simulink model "F16TestHarness"  (R2024a)
settings: configuration reference "standardSILConfiguraitonParams" (kept outside this file)
undefined symbols (not defined in the file): airDensity_kgpm3, Earth, referenceLatitude_deg, referenceLongitude_deg, speedOfSound_mps, terrainHeightNED_m, visualizationType, WGS84
libraries: aerolibtransform2 x2, aerolibatmos2 x1, aerolibfltsims x1, sharedtransform x1, robotcorelib x1, uavutilslib x1
settings Model: Creator=jerem  LastModifiedBy=jerem
settings ConfigSetRef: SourceName=standardSILConfiguraitonParams  SourceLocation=Base Workspace

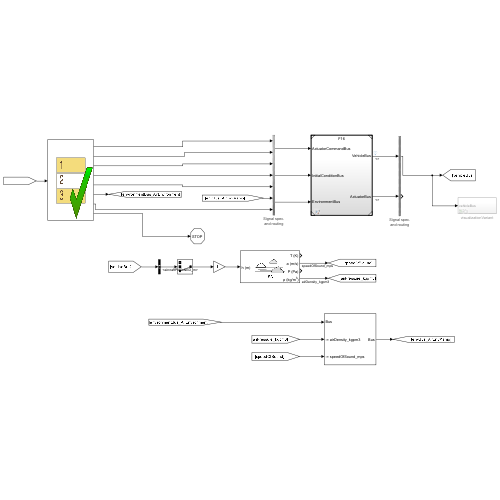
[thumbnail: Simulink's stored preview of the top-level diagram]
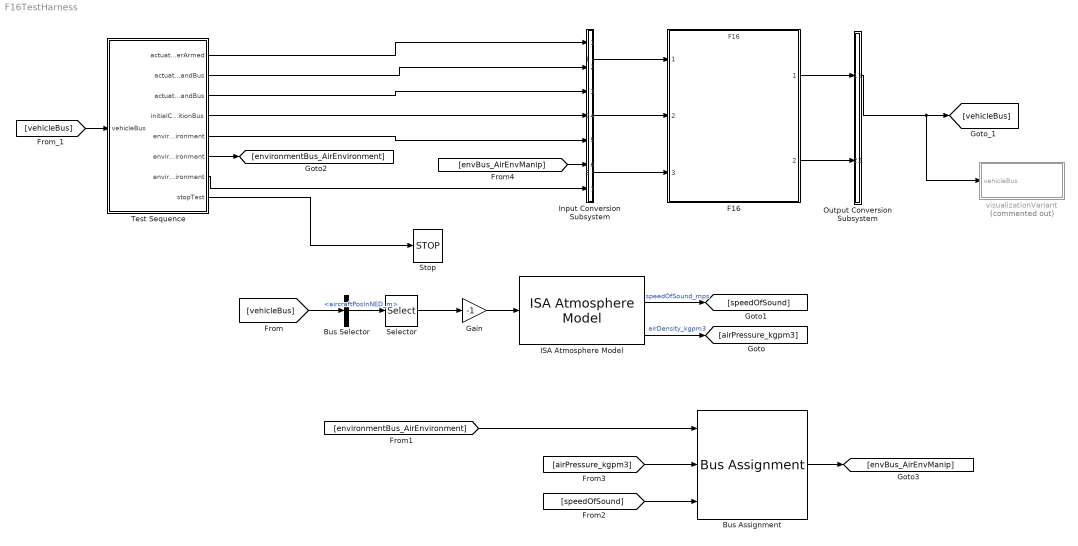
== system F16TestHarness ==
  Bus Assignment : BusAssignment  AssignedSignals=airDensity_kgpm3,speedOfSound_mps
  Bus Selector : BusSelector  OutputSignals=BodyStates.aircraftPosInNED_m
  F16 : ModelReference  ModelNameDialog=F16  SimulationMode=Normal  ModelReferenceVersion=1.92
  Gain : Gain  Gain=-1
  ISA Atmosphere Model : aerolibatmos2/ISA Atmosphere Model  useExtended=off  action=Warning  custom=off  viscosityOut=off  g=9.80665  gamma=1.4  R=287.0531  L=0.0065  h_trop=11000  h_strat=20000  rho0=1.225  P0=101325  T0=288.15  h0=0  S=110.4  Tref=273.15  muref=1.716e-5
  Input Conversion Subsystem : Subsystem  Tag=__SLT_ICS__  Description=|
      | Signal spec.
      | and routing
      settings: AttributesFormatString=%<Description>
  Output Conversion Subsystem : Subsystem  Tag=__SLT_OCS__  Description=|
      | Signal spec.
      | and routing
      mask init:
      | ICDictionary = get_param(bdroot, 'DataDictionary');
      | if isempty(ICDictionary)
      |    ICScope = Simulink.data.BaseWorkspace;
      | else
      |    ICScope = Simulink.data.DataDictionary(ICDictionary);
      | end
      | 
      | IC1 = Simulink.Bus.createMATLABStruct('VehicleBus', [], [1 1], ICScope);
      | IC2 = Simulink.Bus.createMATLABStruct('ActuatorBus', [], [1 1], ICScope);
      settings: AttributesFormatString=%<Description>
  Selector : Selector  InputPortWidth=3  IndexOptions=Index vector (dialog)  Indices=3  OutputSizes=1
  Stop : Stop
  Test Sequence : Test Sequence  TreatAsAtomicUnit=on
  visualizationVariant : Subsystem  Commented=on  Variant=on
  wires:
  Test Sequence/1(actuatorCommandBus_controllerArmed) -> Input Conversion Subsystem/1(Inport_1)
  Test Sequence/2(actuatorCommandBus_ServosCommandBus) -> Input Conversion Subsystem/2(Inport_2)
  Test Sequence/3(actuatorCommandBus_EngineCommandBus) -> Input Conversion Subsystem/3(Inport_3)
  Test Sequence/4(initialConditionBus) -> Input Conversion Subsystem/4(Inport_4)
  Test Sequence/5(environmentBus_EarthEnvironment) -> Input Conversion Subsystem/5(Inport_5)
  Test Sequence/6(environmentBus_AirEnvironment) -> [environmentBus_AirEnvironment]
  Test Sequence/7(environmentBus_TerrainEnvironment) -> Input Conversion Subsystem/7(Inport_7)
  [vehicleBus] -> Test Sequence/1(vehicleBus)
  Output Conversion Subsystem/1(Outport_1) -> visualizationVariant/1(vehicleBus), [vehicleBus]
  Test Sequence/8(stopTest) -> Stop/1
  [vehicleBus] -> Bus Selector/1
  Selector/1 -> Gain/1
  Bus Selector/1 -> Selector/1  "<aircraftPosInNED_m>"
  Gain/1 -> ISA Atmosphere Model/1
  ISA Atmosphere Model/4 -> [airPressure_kgpm3]  "airDensity_kgpm3"
  ISA Atmosphere Model/2 -> [speedOfSound]  "speedOfSound_mps"
  [environmentBus_AirEnvironment] -> Bus Assignment/1
  [speedOfSound] -> Bus Assignment/3
  [airPressure_kgpm3] -> Bus Assignment/2
  Bus Assignment/1 -> [envBus_AirEnvManip]
  [envBus_AirEnvManip] -> Input Conversion Subsystem/6(Inport_6)
  F16/1 -> Output Conversion Subsystem/1(Inport_1)
  F16/2 -> Output Conversion Subsystem/2(Inport_2)
  Input Conversion Subsystem/1(Outport_1) -> F16/1
  Input Conversion Subsystem/2(Outport_2) -> F16/2
  Input Conversion Subsystem/3(Outport_3) -> F16/3

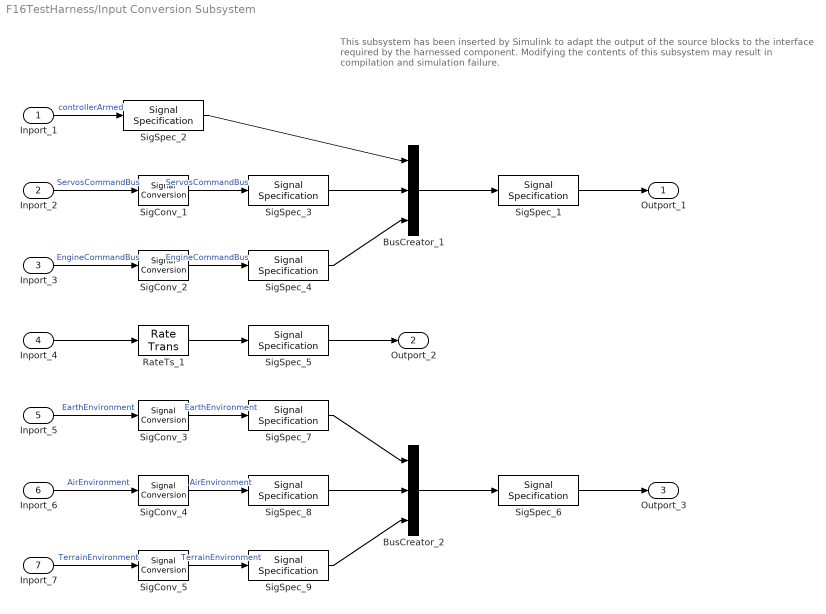
== system F16TestHarness/Input Conversion Subsystem ==
  note: This subsystem has been inserted by Simulink to adapt the output of the source blocks to the interface required by the harnessed component.
      |  Modifying the contents of this subsystem may result in compilation and simulation failure.
  Inport_1 : Inport
  Inport_2 : Inport  Port=2
  Inport_3 : Inport  Port=3
  Inport_4 : Inport  Port=4
  Inport_5 : Inport  Port=5
  Inport_6 : Inport  Port=6
  Inport_7 : Inport  Port=7
  BusCreator_1 : BusCreator  Inputs=3  OutDataTypeStr=Bus: ActuatorCommandBus
  BusCreator_2 : BusCreator  Inputs=3  OutDataTypeStr=Bus: EnvironmentBus
  RateTs_1 : RateTransition  OutPortSampleTime=0.004
  SigConv_{1..5} (5 alike) : SignalConversion  ConversionOutput=Nonvirtual bus  OverrideOpt=off
  SigSpec_1 : SignalSpecification  OutDataTypeStr=Bus: ActuatorCommandBus  SampleTime=[-1, 0]
  SigSpec_2 : SignalSpecification  OutDataTypeStr=double  Dimensions=[1]  SampleTime=[-1, 0]
  SigSpec_3 : SignalSpecification  OutDataTypeStr=Bus: ServosCommandBus  Dimensions=[1]  SampleTime=[-1, 0]  BusOutputAsStruct=on
  SigSpec_4 : SignalSpecification  OutDataTypeStr=Bus: EngineCommandBus  Dimensions=[1]  SampleTime=[-1, 0]  BusOutputAsStruct=on
  SigSpec_5 : SignalSpecification  OutDataTypeStr=double  Dimensions=[1]  SampleTime=0.004
  SigSpec_6 : SignalSpecification  OutDataTypeStr=Bus: EnvironmentBus  SampleTime=[-1, 0]
  SigSpec_7 : SignalSpecification  OutDataTypeStr=Bus: EarthEnvironmentBus  Dimensions=[1]  SampleTime=[-1, 0]  BusOutputAsStruct=on
  SigSpec_8 : SignalSpecification  OutDataTypeStr=Bus: AirEnvironmentBus  Dimensions=[1]  SampleTime=[-1, 0]  BusOutputAsStruct=on
  SigSpec_9 : SignalSpecification  OutDataTypeStr=Bus: TerrainEnvironmentBus  Dimensions=[1]  SampleTime=[-1, 0]  BusOutputAsStruct=on
  Outport_1 : Outport
  Outport_2 : Outport  Port=2
  Outport_3 : Outport  Port=3
  wires:
  SigSpec_1/1 -> Outport_1/1
  BusCreator_1/1 -> SigSpec_1/1
  SigSpec_2/1 -> BusCreator_1/1
  Inport_1/1 -> SigSpec_2/1  "controllerArmed"
  SigSpec_3/1 -> BusCreator_1/2
  SigConv_1/1 -> SigSpec_3/1  "ServosCommandBus"
  Inport_2/1 -> SigConv_1/1  "ServosCommandBus"
  SigSpec_4/1 -> BusCreator_1/3
  SigConv_2/1 -> SigSpec_4/1  "EngineCommandBus"
  Inport_3/1 -> SigConv_2/1  "EngineCommandBus"
  SigSpec_5/1 -> Outport_2/1
  RateTs_1/1 -> SigSpec_5/1
  Inport_4/1 -> RateTs_1/1
  SigSpec_6/1 -> Outport_3/1
  BusCreator_2/1 -> SigSpec_6/1
  SigSpec_7/1 -> BusCreator_2/1
  SigConv_3/1 -> SigSpec_7/1  "EarthEnvironment"
  Inport_5/1 -> SigConv_3/1  "EarthEnvironment"
  SigSpec_8/1 -> BusCreator_2/2
  SigConv_4/1 -> SigSpec_8/1  "AirEnvironment"
  Inport_6/1 -> SigConv_4/1  "AirEnvironment"
  SigSpec_9/1 -> BusCreator_2/3
  SigConv_5/1 -> SigSpec_9/1  "TerrainEnvironment"
  Inport_7/1 -> SigConv_5/1  "TerrainEnvironment"

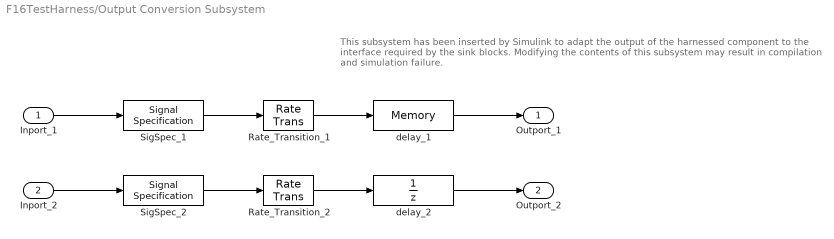
== system F16TestHarness/Output Conversion Subsystem ==
  note: This subsystem has been inserted by Simulink to adapt the output of the harnessed component to the interface required by the sink blocks.
      |  Modifying the contents of this subsystem may result in compilation and simulation failure.
  Inport_1 : Inport
  Inport_2 : Inport  Port=2
  Rate_Transition_1 : RateTransition  OutPortSampleTimeOpt=Inherit
  Rate_Transition_2 : RateTransition  OutPortSampleTimeOpt=Inherit
  SigSpec_1 : SignalSpecification  OutDataTypeStr=Bus: VehicleBus  Dimensions=[1]
  SigSpec_2 : SignalSpecification  OutDataTypeStr=Bus: ActuatorBus  Dimensions=[1]
  delay_1 : Memory  InitialCondition=IC1
  delay_2 : UnitDelay  InitialCondition=IC2  SampleTime=-1
  Outport_1 : Outport
  Outport_2 : Outport  Port=2
  wires:
  Inport_1/1 -> SigSpec_1/1
  SigSpec_1/1 -> Rate_Transition_1/1
  Rate_Transition_1/1 -> delay_1/1
  delay_1/1 -> Outport_1/1
  Inport_2/1 -> SigSpec_2/1
  SigSpec_2/1 -> Rate_Transition_2/1
  Rate_Transition_2/1 -> delay_2/1
  delay_2/1 -> Outport_2/1

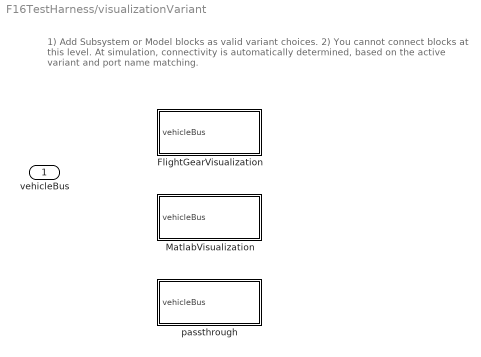
== system F16TestHarness/visualizationVariant ==
  note: 1) Add Subsystem or Model blocks as valid variant choices.
      | 2) You cannot connect blocks at this level. At simulation, connectivity is automatically
      | determined, based on the active variant and port name matching.
  vehicleBus : Inport
  FlightGearVisualization : Subsystem  TreatAsAtomicUnit=on  VariantControl="strcmp(visualizationType, \"FlightGear\")"
  MatlabVisualization : Subsystem  VariantControl="strcmp(visualizationType, \"Matlab\")"
  passthrough : Subsystem  VariantControl="strcmp(visualizationType, \"PassThrough\")"

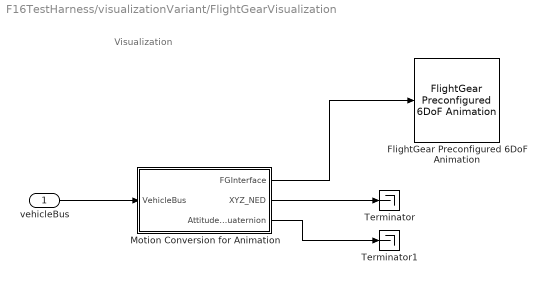
== system F16TestHarness/visualizationVariant/FlightGearVisualization ==
  note: Visualization
  vehicleBus : Inport
  FlightGear Preconfigured 6DoF Animation : aerolibfltsims/FlightGear Preconfigured 6DoF Animation  xFlightGearVersion=v2019.1  DestinationIpAddress=127.0.0.1  DestinationPort=5502  SampleTime=-1  packetVersion=24
  Motion Conversion for Animation : Subsystem
      mask Display:
      | port_label('input',1,'ACBus')
      | port_label('output',1,'\lambda,L,h,\phi,\theta,\psi','texmode','on')
  Terminator : Terminator
  Terminator1 : Terminator
  wires:
  Motion Conversion for Animation/1(FGInterface) -> FlightGear Preconfigured 6DoF Animation/1
  vehicleBus/1 -> Motion Conversion for Animation/1(VehicleBus)
  Motion Conversion for Animation/2(XYZ_NED) -> Terminator/1
  Motion Conversion for Animation/3(AttitudeQuaternion) -> Terminator1/1

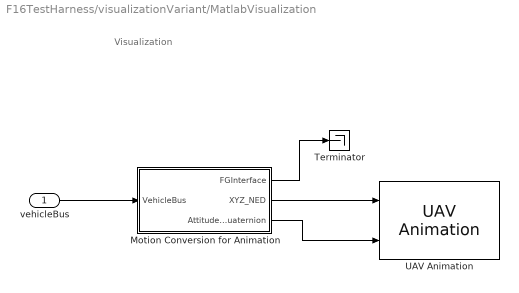
== system F16TestHarness/visualizationVariant/MatlabVisualization ==
  note: Visualization
  vehicleBus : Inport
  Motion Conversion for Animation : Subsystem
      mask Display:
      | port_label('input',1,'ACBus')
      | port_label('output',1,'\lambda,L,h,\phi,\theta,\psi','texmode','on')
  Terminator : Terminator
  UAV Animation : uavutilslib/UAV Animation  UAVType=FixedWing  UAVSize=100  InertialZDirection=Down  SampleTime=-1
  wires:
  Motion Conversion for Animation/2(XYZ_NED) -> UAV Animation/1
  vehicleBus/1 -> Motion Conversion for Animation/1(VehicleBus)
  Motion Conversion for Animation/3(AttitudeQuaternion) -> UAV Animation/2
  Motion Conversion for Animation/1(FGInterface) -> Terminator/1

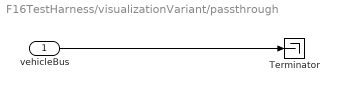
== system F16TestHarness/visualizationVariant/passthrough ==
  vehicleBus : Inport
  Terminator : Terminator
  wires:
  vehicleBus/1 -> Terminator/1

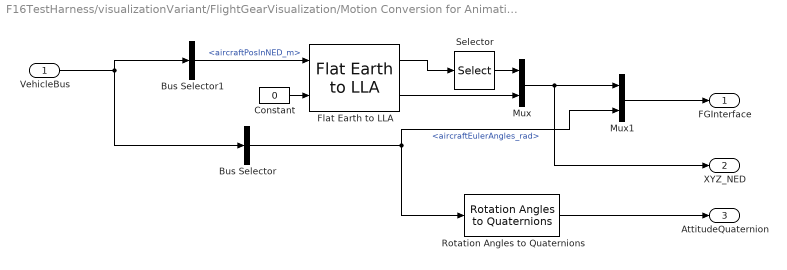
== system F16TestHarness/visualizationVariant/FlightGearVisualization/Motion Conversion for Animation ==
  VehicleBus : Inport  OutDataTypeStr=Bus: VehicleBus
  Bus Selector : BusSelector  OutputSignals=BodyStates.aircraftEulerAngles_rad
  Bus Selector1 : BusSelector  OutputSignals=BodyStates.aircraftPosInNED_m
  Constant : Constant  Value=0
  Flat Earth to LLA : aerolibtransform2/Flat Earth to LLA  units=Metric (MKS)  ptype=Earth (WGS84)  F=1/298.257223563  R=6378137  refPosPort=off  LL0=[referenceLatitude_deg, referenceLongitude_deg]  psi=0
  Mux : Mux  Inputs=2
  Mux1 : Mux  Inputs=2
  Rotation Angles to Quaternions : sharedtransform/Rotation Angles to Quaternions  rotationOrder=ZYX  aMode=aMode
  Selector : Selector  IndexMode=Zero-based  InputPortWidth=2  IndexOptions=Index vector (dialog)  Indices=[1 0]  OutputSizes=1
  FGInterface : Outport  VectorParamsAs1DForOutWhenUnconnected=off
  XYZ_NED : Outport  Port=2  VectorParamsAs1DForOutWhenUnconnected=off
  AttitudeQuaternion : Outport  Port=3  VectorParamsAs1DForOutWhenUnconnected=off
  wires:
  Mux1/1 -> FGInterface/1
  Constant/1 -> Flat Earth to LLA/2
  Bus Selector/1 -> Rotation Angles to Quaternions/1, Mux1/2  "<aircraftEulerAngles_rad>"
  Flat Earth to LLA/2 -> Mux/2
  Flat Earth to LLA/1 -> Selector/1
  Bus Selector1/1 -> Flat Earth to LLA/1  "<aircraftPosInNED_m>"
  VehicleBus/1 -> Bus Selector/1, Bus Selector1/1
  Selector/1 -> Mux/1
  Mux/1 -> XYZ_NED/1, Mux1/1
  Rotation Angles to Quaternions/1 -> AttitudeQuaternion/1

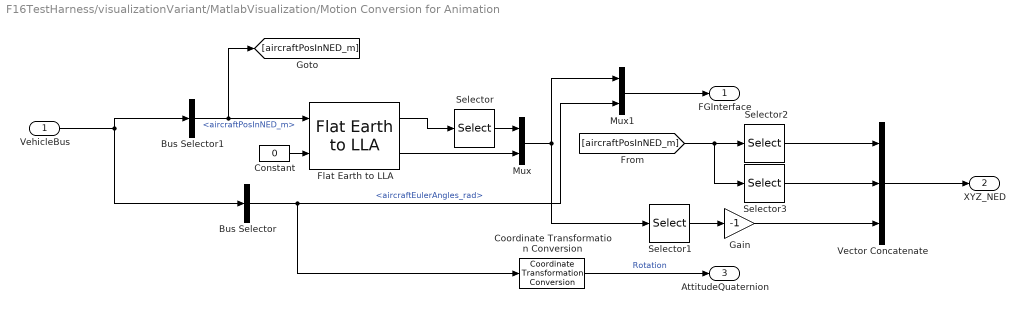
== system F16TestHarness/visualizationVariant/MatlabVisualization/Motion Conversion for Animation ==
  VehicleBus : Inport  OutDataTypeStr=Bus: VehicleBus
  Bus Selector : BusSelector  OutputSignals=BodyStates.aircraftEulerAngles_rad
  Bus Selector1 : BusSelector  OutputSignals=BodyStates.aircraftPosInNED_m
  Constant : Constant  Value=0
  Coordinate Transformation Conversion : robotcorelib/Coordinate Transformation Conversion  InputRepresentation=Euler Angles  InputEulerSequence=XYZ  ShowTrVecInputPort=on  OutputRepresentation=Quaternion  OutputEulerSequence=ZYX  ShowTrVecOutputPort=on  SimulateUsing=Code generation
  Flat Earth to LLA : aerolibtransform2/Flat Earth to LLA  units=Metric (MKS)  ptype=Earth (WGS84)  F=1/298.257223563  R=6378137  refPosPort=off  LL0=[referenceLatitude_deg, referenceLongitude_deg]  psi=0
  Gain : Gain  Gain=-1
  Mux : Mux  Inputs=2
  Mux1 : Mux  Inputs=2
  Selector : Selector  IndexMode=Zero-based  InputPortWidth=2  IndexOptions=Index vector (dialog)  Indices=[1 0]  OutputSizes=1
  Selector1 : Selector  InputPortWidth=3  IndexOptions=Index vector (dialog)  Indices=3  OutputSizes=1
  Selector2 : Selector  InputPortWidth=3  IndexOptions=Index vector (dialog)  Indices=1  OutputSizes=1
  Selector3 : Selector  InputPortWidth=3  IndexOptions=Index vector (dialog)  Indices=2  OutputSizes=1
  Vector Concatenate : Concatenate  NumInputs=3
  FGInterface : Outport  VectorParamsAs1DForOutWhenUnconnected=off
  XYZ_NED : Outport  Port=2  VectorParamsAs1DForOutWhenUnconnected=off
  AttitudeQuaternion : Outport  Port=3  VectorParamsAs1DForOutWhenUnconnected=off
  wires:
  Mux1/1 -> FGInterface/1
  Constant/1 -> Flat Earth to LLA/2
  Bus Selector/1 -> Coordinate Transformation Conversion/1, Mux1/2  "<aircraftEulerAngles_rad>"
  Flat Earth to LLA/2 -> Mux/2
  Flat Earth to LLA/1 -> Selector/1
  Bus Selector1/1 -> [aircraftPosInNED_m], Flat Earth to LLA/1  "<aircraftPosInNED_m>"
  VehicleBus/1 -> Bus Selector/1, Bus Selector1/1
  Selector/1 -> Mux/1
  Mux/1 -> Selector1/1, Mux1/1
  Selector2/1 -> Vector Concatenate/1
  Selector3/1 -> Vector Concatenate/2
  Vector Concatenate/1 -> XYZ_NED/1
  Selector1/1 -> Gain/1
  Gain/1 -> Vector Concatenate/3
  [aircraftPosInNED_m] -> Selector3/1, Selector2/1
  Coordinate Transformation Conversion/1 -> AttitudeQuaternion/1  "Rotation"

== stateflow chart F16TestHarness/Test Sequence ==
  state Scenario_1
    state Initialize
      %% Initialize data outputs.
      actuatorCommandBus_controllerArmed = 0;
      actuatorCommandBus_ServosCommandBus.ServosCommandF16Bus.cmdAileron_nd = 0;
      actuatorCommandBus_ServosCommandBus.ServosCommandF16Bus.cmdElevator_nd = 0;
      actuatorCommandBus_ServosCommandBus.ServosCommandF16Bus.cmdRudder_nd = 0;
      actuatorCommandBus_EngineCommandBus.cmdThrottle_unit = 0;
      initialConditionBus = 0;
      environmentBus_EarthEnvironment.gravityScalar_mps2 = 9.80665;
      environmentBus_EarthEnvironment.worldMagneticFieldInNED_nT = zeros(3,1);
      environmentBus_AirEnvironment.airTemperature_K = 0;
      environmentBus_AirEnvironment.airPressure_Pa = 0;
      environmentBus_AirEnvironment.airDensity_kgpm3 = 1.225;
      environmentBus_AirEnvironment.windSpeedInNED_mps = zeros(3,1);
      environmentBus_AirEnvironment.speedOfSound_mps = 0;
      environmentBus_AirEnvironment.windsAloftInNED_mps = zeros(3,1);
      environmentBus_AirEnvironment.gustInNED_mps = zeros(3,1);
      environmentBus_AirEnvironment.turbulenceInNED_mps = zeros(3,1);
      environmentBus_TerrainEnvironment.terrainHeightInNED_m = terrainHeightNED_m;
      stopTest = false;
    state verifyZeroInputs
      verify(isClose(vehicleBus.AircraftForcesMoments.forcesInBody_N(1), 0 ))
      verify(isClose(vehicleBus.AircraftForcesMoments.forcesInBody_N(2), 0 ))
      verify(isClose(vehicleBus.AircraftForcesMoments.forcesInBody_N(3), 0 ))
      verify(isClose(vehicleBus.AircraftForcesMoments.momentsInBody_Nm(1),0))
      verify(isClose(vehicleBus.AircraftForcesMoments.momentsInBody_Nm(2),0))
      verify(isClose(vehicleBus.AircraftForcesMoments.momentsInBody_Nm(3),0))
    state throttleNoArm
      actuatorCommandBus_EngineCommandBus.cmdThrottle_unit = 0.1;
    state noThrottleArm
      actuatorCommandBus_controllerArmed = 1;
      actuatorCommandBus_EngineCommandBus.cmdThrottle_unit = 0.0;
      %actuatorCommandBus_ServosCommandBus.ServosCommandF16Bus.cmdElevator_nd = -0.1;
    state verifyZeroInputsAgain
      verify(isClose(vehicleBus.AircraftForcesMoments.forcesInBody_N(1), 0 ))
      verify(isClose(vehicleBus.AircraftForcesMoments.forcesInBody_N(2), 0 ))
      verify(isClose(vehicleBus.AircraftForcesMoments.forcesInBody_N(3), 0 ))
      verify(isClose(vehicleBus.AircraftForcesMoments.momentsInBody_Nm(1),0))
      verify(isClose(vehicleBus.AircraftForcesMoments.momentsInBody_Nm(2),0))
      verify(isClose(vehicleBus.AircraftForcesMoments.momentsInBody_Nm(3),0))
    state armedAndSmallThrottle
      actuatorCommandBus_EngineCommandBus.cmdThrottle_unit = 0.25;
    state verifyThrottle
      verify(vehicleBus.AircraftForcesMoments.forcesInBody_N(1) > 0)
      verify(isClose(vehicleBus.AircraftForcesMoments.forcesInBody_N(2), 0 ))
      verify(isClose(vehicleBus.AircraftForcesMoments.forcesInBody_N(3), 0 ))
      verify(isClose(vehicleBus.AircraftForcesMoments.momentsInBody_Nm(1),0))
      verify(isClose(vehicleBus.AircraftForcesMoments.momentsInBody_Nm(2),0))
      verify(isClose(vehicleBus.AircraftForcesMoments.momentsInBody_Nm(3),0))
    state deflectElevatorCreatingNegPitch
      actuatorCommandBus_ServosCommandBus.ServosCommandF16Bus.cmdElevator_nd = 0.25;
      actuatorCommandBus_EngineCommandBus.cmdThrottle_unit = 0.75;
    state verifyPitchIntoGround
      verify(isClose(vehicleBus.AircraftForcesMoments.momentsInBody_Nm(2), 0))
      verify(isClose(vehicleBus.BodyStates.aircraftEulerAngles_rad(2) , 0))
      verify(isClose(vehicleBus.AircraftForcesMoments.forcesInBody_N(3), 0))
      verify(vehicleBus.AircraftForcesMoments.forcesInBody_N(1) > 0)
      verify(isClose(vehicleBus.AircraftForcesMoments.forcesInBody_N(2), 0 ))
    state deflectElevator
      actuatorCommandBus_ServosCommandBus.ServosCommandF16Bus.cmdElevator_nd = -0.025;
      actuatorCommandBus_EngineCommandBus.cmdThrottle_unit = 1;
    state verifydeflectElevator
      verify(isClose(vehicleBus.AircraftForcesMoments.momentsInBody_Nm(2), 0, 'absTol', 0.01)) % Shouldn't be enough elevator to rotate vehicle
      verify(isClose(vehicleBus.BodyStates.aircraftEulerAngles_rad(2), 0, 'absTol', 0.01 )) % Shouldn't be enough elevator to rotate vehicle
      verify(isClose(vehicleBus.AircraftForcesMoments.forcesInBody_N(3), 0, 'absTol', 0.01))
      verify(vehicleBus.AircraftForcesMoments.forcesInBody_N(1) > 0)
      verify(isClose(vehicleBus.AircraftForcesMoments.forcesInBody_N(2), 0 ))
    state rotate
      actuatorCommandBus_ServosCommandBus.ServosCommandF16Bus.cmdElevator_nd = -0.08;
    state verifyRotate
      verify(vehicleBus.AircraftForcesMoments.momentsInBody_Nm(2) > 0)
      verify(vehicleBus.BodyStates.aircraftEulerAngles_rad(2) > 0)
      verify(vehicleBus.AircraftForcesMoments.forcesInBody_N(3) < 0)
      verify(vehicleBus.AircraftForcesMoments.forcesInBody_N(1) > 0)
      verify(isClose(vehicleBus.AircraftForcesMoments.forcesInBody_N(2), 0 ))
    state continueFlying
      actuatorCommandBus_ServosCommandBus.ServosCommandF16Bus.cmdElevator_nd = -0.04;
      actuatorCommandBus_EngineCommandBus.cmdThrottle_unit = 1;
    state verifyFlying
      verify(vehicleBus.BodyStates.aircraftPosInNED_m(3) < 0)
      verify(vehicleBus.BodyStates.aircraftEulerAngles_rad(2) > 0)
      verify(vehicleBus.AircraftForcesMoments.forcesInBody_N(1) > 0)
      verify(isClose(vehicleBus.AircraftForcesMoments.forcesInBody_N(2), 0 ))
    state EndTest
      stopTest = true;
    (default) -> Scenario_1.Initialize
    Scenario_1.Initialize -> verifyZeroInputs : [
        | after(1,tick)
        | ]
    verifyZeroInputs -> throttleNoArm : [
        | after(5,sec)
        | ]
    throttleNoArm -> noThrottleArm : [
        | after(1,sec)
        | ]
    noThrottleArm -> verifyZeroInputsAgain : [
        | after(3,sec)
        | ]
    verifyZeroInputsAgain -> armedAndSmallThrottle : [
        | after(5,sec)
        | ]
    armedAndSmallThrottle -> verifyThrottle : [
        | after(60,sec)
        | ]
    verifyThrottle -> deflectElevatorCreatingNegPitch : [
        | after(1,tick)
        | ]
    deflectElevatorCreatingNegPitch -> verifyPitchIntoGround : [
        | after(3,sec)
        | ]
    verifyPitchIntoGround -> deflectElevator : [
        | after(1,sec)
        | ]
    deflectElevator -> verifydeflectElevator : [
        | after(2,sec)
        | ]
    verifydeflectElevator -> rotate : [
        | after(1,tick)
        | ]
    rotate -> verifyRotate : [
        | after(3,sec)
        | ]
    verifyRotate -> continueFlying : [
        | after(1,tick)
        | ]
    continueFlying -> verifyFlying : [
        | after(3,sec)
        | ]
    verifyFlying -> Scenario_1.EndTest : [
        | after(1,tick)
        | ]
  state SameAsVehiclePlantHarness
    state Initialize
      %% Initialize data outputs.
      actuatorCommandBus_controllerArmed = 0;
      actuatorCommandBus_ServosCommandBus.ServosCommandF16Bus.cmdAileron_nd = 0;
      actuatorCommandBus_ServosCommandBus.ServosCommandF16Bus.cmdElevator_nd = 0;
      actuatorCommandBus_ServosCommandBus.ServosCommandF16Bus.cmdRudder_nd = 0;
      actuatorCommandBus_EngineCommandBus.cmdThrottle_unit = 0;
      initialConditionBus = 0;
      environmentBus_EarthEnvironment.gravityScalar_mps2 = 9.80665;
      environmentBus_EarthEnvironment.worldMagneticFieldInNED_nT = zeros(3,1);
      environmentBus_AirEnvironment.airTemperature_K = 0;
      environmentBus_AirEnvironment.airPressure_Pa = 0;
      environmentBus_AirEnvironment.airDensity_kgpm3 = 1.225;
      environmentBus_AirEnvironment.windSpeedInNED_mps = zeros(3,1);
      environmentBus_AirEnvironment.speedOfSound_mps = 0;
      environmentBus_AirEnvironment.windsAloftInNED_mps = zeros(3,1);
      environmentBus_AirEnvironment.gustInNED_mps = zeros(3,1);
      environmentBus_AirEnvironment.turbulenceInNED_mps = zeros(3,1);
      environmentBus_TerrainEnvironment.terrainHeightInNED_m = terrainHeightNED_m;
      stopTest = false;
    state step_1
      actuatorCommandBus_controllerArmed = 1;
      actuatorCommandBus_ServosCommandBus.ServosCommandF16Bus.cmdElevator_nd = -0.15;
      actuatorCommandBus_EngineCommandBus.cmdThrottle_unit = 1;
    state step_2
      actuatorCommandBus_ServosCommandBus.ServosCommandF16Bus.cmdElevator_nd  = -0.03;
    state step_3
      actuatorCommandBus_ServosCommandBus.ServosCommandF16Bus.cmdElevator_nd  = -0.1;
    state EndTest
      stopTest = true;
    (default) -> SameAsVehiclePlantHarness.Initialize
    SameAsVehiclePlantHarness.Initialize -> SameAsVehiclePlantHarness.step_1 : [
        | after(1,tick)
        | ]
    SameAsVehiclePlantHarness.step_1 -> SameAsVehiclePlantHarness.step_2 : [
        | after(30,sec)
        | ]
    SameAsVehiclePlantHarness.step_2 -> SameAsVehiclePlantHarness.step_3 : [
        | after(100,sec)
        | ]
    SameAsVehiclePlantHarness.step_3 -> SameAsVehiclePlantHarness.EndTest : [
        | after(150,sec)
        | ]
  state MaxAirspeedTest
    state Initialize
      %% Initialize data outputs.
      actuatorCommandBus_controllerArmed = 0;
      actuatorCommandBus_ServosCommandBus.ServosCommandF16Bus.cmdAileron_nd = 0;
      actuatorCommandBus_ServosCommandBus.ServosCommandF16Bus.cmdElevator_nd = 0;
      actuatorCommandBus_ServosCommandBus.ServosCommandF16Bus.cmdRudder_nd = 0;
      actuatorCommandBus_EngineCommandBus.cmdThrottle_unit = 0;
      initialConditionBus = 0;
      environmentBus_EarthEnvironment.gravityScalar_mps2 = 9.80665;
      environmentBus_EarthEnvironment.worldMagneticFieldInNED_nT = zeros(3,1);
      environmentBus_AirEnvironment.airTemperature_K = 0;
      environmentBus_AirEnvironment.airPressure_Pa = 0;
      environmentBus_AirEnvironment.airDensity_kgpm3 = 1.225;
      environmentBus_AirEnvironment.windSpeedInNED_mps = zeros(3,1);
      environmentBus_AirEnvironment.speedOfSound_mps = 0;
      environmentBus_AirEnvironment.windsAloftInNED_mps = zeros(3,1);
      environmentBus_AirEnvironment.gustInNED_mps = zeros(3,1);
      environmentBus_AirEnvironment.turbulenceInNED_mps = zeros(3,1);
      environmentBus_TerrainEnvironment.terrainHeightInNED_m = terrainHeightNED_m;
      stopTest = false;
    state step_1
      actuatorCommandBus_controllerArmed = 1;
      actuatorCommandBus_ServosCommandBus.ServosCommandF16Bus.cmdElevator_nd = -0.05;
      actuatorCommandBus_EngineCommandBus.cmdThrottle_unit = 1;
    state step_2
      actuatorCommandBus_ServosCommandBus.ServosCommandF16Bus.cmdElevator_nd = 0;
    state EndTest
      stopTest = true;
    (default) -> MaxAirspeedTest.Initialize
    MaxAirspeedTest.Initialize -> MaxAirspeedTest.step_1 : [
        | after(1,tick)
        | ]
    MaxAirspeedTest.step_1 -> MaxAirspeedTest.step_2 : [
        | after(25,sec)
        | ]
    MaxAirspeedTest.step_2 -> MaxAirspeedTest.EndTest : [
        | after(200,sec)
        | ]
  state TakeoffLevelFlight
    state Initialize
      %% Initialize data outputs.
      actuatorCommandBus_controllerArmed = 0;
      actuatorCommandBus_ServosCommandBus.ServosCommandF16Bus.cmdAileron_nd = 0;
      actuatorCommandBus_ServosCommandBus.ServosCommandF16Bus.cmdElevator_nd = 0;
      actuatorCommandBus_ServosCommandBus.ServosCommandF16Bus.cmdRudder_nd = 0;
      actuatorCommandBus_EngineCommandBus.cmdThrottle_unit = 0;
      initialConditionBus = 0;
      environmentBus_EarthEnvironment.gravityScalar_mps2 = 9.80665;
      environmentBus_EarthEnvironment.worldMagneticFieldInNED_nT = zeros(3,1);
      environmentBus_AirEnvironment.airTemperature_K = 0;
      environmentBus_AirEnvironment.airPressure_Pa = 0;
      environmentBus_AirEnvironment.airDensity_kgpm3 = 1.225;
      environmentBus_AirEnvironment.windSpeedInNED_mps = zeros(3,1);
      environmentBus_AirEnvironment.speedOfSound_mps = 0;
      environmentBus_AirEnvironment.windsAloftInNED_mps = zeros(3,1);
      environmentBus_AirEnvironment.gustInNED_mps = zeros(3,1);
      environmentBus_AirEnvironment.turbulenceInNED_mps = zeros(3,1);
      environmentBus_TerrainEnvironment.terrainHeightInNED_m = terrainHeightNED_m;
      stopTest = false;
    state step_2
      actuatorCommandBus_controllerArmed = 1;
      actuatorCommandBus_EngineCommandBus.cmdThrottle_unit = 1;
    state step_3
      actuatorCommandBus_ServosCommandBus.ServosCommandF16Bus.cmdElevator_nd = -0.08;
    state step_1
      actuatorCommandBus_ServosCommandBus.ServosCommandF16Bus.cmdElevator_nd = -0.04;
    state step_4
      actuatorCommandBus_ServosCommandBus.ServosCommandF16Bus.cmdElevator_nd = -0.028;
    state EndTest
      stopTest = true;
    (default) -> TakeoffLevelFlight.Initialize
    TakeoffLevelFlight.Initialize -> TakeoffLevelFlight.step_2 : [
        | after(1,tick)
        | ]
    TakeoffLevelFlight.step_2 -> TakeoffLevelFlight.step_3 : [
        | after(22,sec)
        | ]
    TakeoffLevelFlight.step_3 -> TakeoffLevelFlight.step_1 : [
        | after(10,sec)
        | ]
    TakeoffLevelFlight.step_1 -> TakeoffLevelFlight.step_4 : [
        | after(20,sec)
        | ]
    TakeoffLevelFlight.step_4 -> TakeoffLevelFlight.EndTest : [
        | after(20,sec)
        | ]
  state pitchTest
    state Initialize
      %% Initialize data outputs.
      actuatorCommandBus_controllerArmed = 0;
      actuatorCommandBus_ServosCommandBus.ServosCommandF16Bus.cmdAileron_nd = 0;
      actuatorCommandBus_ServosCommandBus.ServosCommandF16Bus.cmdElevator_nd = 0;
      actuatorCommandBus_ServosCommandBus.ServosCommandF16Bus.cmdRudder_nd = 0;
      actuatorCommandBus_EngineCommandBus.cmdThrottle_unit = 0;
      initialConditionBus = 0;
      environmentBus_EarthEnvironment.gravityScalar_mps2 = 9.80665;
      environmentBus_EarthEnvironment.worldMagneticFieldInNED_nT = zeros(3,1);
      environmentBus_AirEnvironment.airTemperature_K = 0;
      environmentBus_AirEnvironment.airPressure_Pa = 0;
      environmentBus_AirEnvironment.airDensity_kgpm3 = 1.225;
      environmentBus_AirEnvironment.windSpeedInNED_mps = zeros(3,1);
      environmentBus_AirEnvironment.speedOfSound_mps = 0;
      environmentBus_AirEnvironment.windsAloftInNED_mps = zeros(3,1);
      environmentBus_AirEnvironment.gustInNED_mps = zeros(3,1);
      environmentBus_AirEnvironment.turbulenceInNED_mps = zeros(3,1);
      environmentBus_TerrainEnvironment.terrainHeightInNED_m = terrainHeightNED_m;
      stopTest = false;
    state step_2
      actuatorCommandBus_controllerArmed = 1;
      actuatorCommandBus_EngineCommandBus.cmdThrottle_unit = 1;
    state step_3
      actuatorCommandBus_ServosCommandBus.ServosCommandF16Bus.cmdElevator_nd = -0.08;
    state step_1
      actuatorCommandBus_ServosCommandBus.ServosCommandF16Bus.cmdElevator_nd = -0.04;
    state step_5
      actuatorCommandBus_ServosCommandBus.ServosCommandF16Bus.cmdElevator_nd = -1;
    state EndTest
      stopTest = true;
    (default) -> pitchTest.Initialize
    pitchTest.Initialize -> pitchTest.step_2 : [
        | after(1,tick)
        | ]
    pitchTest.step_2 -> pitchTest.step_3 : [
        | after(22,sec)
        | ]
    pitchTest.step_3 -> pitchTest.step_1 : [
        | after(10,sec)
        | ]
    pitchTest.step_5 -> pitchTest.EndTest : [
        | after(8,sec)
        | ]
    pitchTest.step_1 -> pitchTest.step_5 : [
        | after(20,sec)
        | ]
  state rollTest
    state Initialize
      %% Initialize data outputs.
      actuatorCommandBus_controllerArmed = 0;
      actuatorCommandBus_ServosCommandBus.ServosCommandF16Bus.cmdAileron_nd = 0;
      actuatorCommandBus_ServosCommandBus.ServosCommandF16Bus.cmdElevator_nd = 0;
      actuatorCommandBus_ServosCommandBus.ServosCommandF16Bus.cmdRudder_nd = 0;
      actuatorCommandBus_EngineCommandBus.cmdThrottle_unit = 0;
      initialConditionBus = 0;
      environmentBus_EarthEnvironment.gravityScalar_mps2 = 9.80665;
      environmentBus_EarthEnvironment.worldMagneticFieldInNED_nT = zeros(3,1);
      environmentBus_AirEnvironment.airTemperature_K = 0;
      environmentBus_AirEnvironment.airPressure_Pa = 0;
      environmentBus_AirEnvironment.airDensity_kgpm3 = 1.225;
      environmentBus_AirEnvironment.windSpeedInNED_mps = zeros(3,1);
      environmentBus_AirEnvironment.speedOfSound_mps = 0;
      environmentBus_AirEnvironment.windsAloftInNED_mps = zeros(3,1);
      environmentBus_AirEnvironment.gustInNED_mps = zeros(3,1);
      environmentBus_AirEnvironment.turbulenceInNED_mps = zeros(3,1);
      environmentBus_TerrainEnvironment.terrainHeightInNED_m = terrainHeightNED_m;
      stopTest = false;
    state step_2
      actuatorCommandBus_controllerArmed = 1;
      actuatorCommandBus_EngineCommandBus.cmdThrottle_unit = 1;
    state step_3
      actuatorCommandBus_ServosCommandBus.ServosCommandF16Bus.cmdElevator_nd = -0.08;
    state step_1
      actuatorCommandBus_ServosCommandBus.ServosCommandF16Bus.cmdElevator_nd = -0.04;
    state step_5
      actuatorCommandBus_ServosCommandBus.ServosCommandF16Bus.cmdAileron_nd= -1;
      actuatorCommandBus_ServosCommandBus.ServosCommandF16Bus.cmdElevator_nd = 0;
    state EndTest
      stopTest = true;
    (default) -> rollTest.Initialize
    rollTest.Initialize -> rollTest.step_2 : [
        | after(1,tick)
        | ]
    rollTest.step_2 -> rollTest.step_3 : [
        | after(22,sec)
        | ]
    rollTest.step_3 -> rollTest.step_1 : [
        | after(10,sec)
        | ]
    rollTest.step_5 -> rollTest.EndTest : [
        | after(2,sec)
        | ]
    rollTest.step_1 -> rollTest.step_5 : [
        | after(20,sec)
        | ]
  state pitchStepInput
    state Initialize
      %% Initialize data outputs.
      actuatorCommandBus_controllerArmed = 0;
      actuatorCommandBus_ServosCommandBus.ServosCommandF16Bus.cmdAileron_nd = 0;
      actuatorCommandBus_ServosCommandBus.ServosCommandF16Bus.cmdElevator_nd = 0;
      actuatorCommandBus_ServosCommandBus.ServosCommandF16Bus.cmdRudder_nd = 0;
      actuatorCommandBus_EngineCommandBus.cmdThrottle_unit = 0;
      initialConditionBus = 0;
      environmentBus_EarthEnvironment.gravityScalar_mps2 = 9.80665;
      environmentBus_EarthEnvironment.worldMagneticFieldInNED_nT = zeros(3,1);
      environmentBus_AirEnvironment.airTemperature_K = 0;
      environmentBus_AirEnvironment.airPressure_Pa = 0;
      environmentBus_AirEnvironment.airDensity_kgpm3 = 1.225;
      environmentBus_AirEnvironment.windSpeedInNED_mps = zeros(3,1);
      environmentBus_AirEnvironment.speedOfSound_mps = 0;
      environmentBus_AirEnvironment.windsAloftInNED_mps = zeros(3,1);
      environmentBus_AirEnvironment.gustInNED_mps = zeros(3,1);
      environmentBus_AirEnvironment.turbulenceInNED_mps = zeros(3,1);
      environmentBus_TerrainEnvironment.terrainHeightInNED_m = terrainHeightNED_m;
      stopTest = false;
    state step_2
      actuatorCommandBus_controllerArmed = 1;
      actuatorCommandBus_EngineCommandBus.cmdThrottle_unit = 1;
    state step_3
      actuatorCommandBus_ServosCommandBus.ServosCommandF16Bus.cmdElevator_nd = -0.08;
    state step_1
      actuatorCommandBus_ServosCommandBus.ServosCommandF16Bus.cmdElevator_nd = -0.06;
    state step_4
      actuatorCommandBus_ServosCommandBus.ServosCommandF16Bus.cmdElevator_nd = -0.028;
    state step_5
      actuatorCommandBus_ServosCommandBus.ServosCommandF16Bus.cmdElevator_nd = -1;
    state step_6
      actuatorCommandBus_ServosCommandBus.ServosCommandF16Bus.cmdElevator_nd = 0;
    state EndTest
      stopTest = true;
    (default) -> pitchStepInput.Initialize
    pitchStepInput.Initialize -> pitchStepInput.step_2 : [
        | after(1,tick)
        | ]
    pitchStepInput.step_2 -> pitchStepInput.step_3 : [
        | after(22,sec)
        | ]
    pitchStepInput.step_3 -> pitchStepInput.step_1 : [
        | after(10,sec)
        | ]
    pitchStepInput.step_1 -> pitchStepInput.step_4 : [
        | after(20,sec)
        | ]
    pitchStepInput.step_4 -> pitchStepInput.step_5 : [
        | after(20,sec)
        | ]
    pitchStepInput.step_5 -> pitchStepInput.step_6 : [
        | after(1,sec)
        | ]
    pitchStepInput.step_6 -> pitchStepInput.EndTest : [
        | after(10,sec)
        | ]
  state rollStepInput
    state Initialize
      %% Initialize data outputs.
      actuatorCommandBus_controllerArmed = 0;
      actuatorCommandBus_ServosCommandBus.ServosCommandF16Bus.cmdAileron_nd = 0;
      actuatorCommandBus_ServosCommandBus.ServosCommandF16Bus.cmdElevator_nd = 0;
      actuatorCommandBus_ServosCommandBus.ServosCommandF16Bus.cmdRudder_nd = 0;
      actuatorCommandBus_EngineCommandBus.cmdThrottle_unit = 0;
      initialConditionBus = 0;
      environmentBus_EarthEnvironment.gravityScalar_mps2 = 9.80665;
      environmentBus_EarthEnvironment.worldMagneticFieldInNED_nT = zeros(3,1);
      environmentBus_AirEnvironment.airTemperature_K = 0;
      environmentBus_AirEnvironment.airPressure_Pa = 0;
      environmentBus_AirEnvironment.airDensity_kgpm3 = 1.225;
      environmentBus_AirEnvironment.windSpeedInNED_mps = zeros(3,1);
      environmentBus_AirEnvironment.speedOfSound_mps = 0;
      environmentBus_AirEnvironment.windsAloftInNED_mps = zeros(3,1);
      environmentBus_AirEnvironment.gustInNED_mps = zeros(3,1);
      environmentBus_AirEnvironment.turbulenceInNED_mps = zeros(3,1);
      environmentBus_TerrainEnvironment.terrainHeightInNED_m = terrainHeightNED_m;
      stopTest = false;
    state step_2
      actuatorCommandBus_controllerArmed = 1;
      actuatorCommandBus_EngineCommandBus.cmdThrottle_unit = 1;
    state step_3
      actuatorCommandBus_ServosCommandBus.ServosCommandF16Bus.cmdElevator_nd = -0.08;
    state step_1
      actuatorCommandBus_ServosCommandBus.ServosCommandF16Bus.cmdElevator_nd = -0.04;
    state step_5
      actuatorCommandBus_ServosCommandBus.ServosCommandF16Bus.cmdAileron_nd= -1;
      actuatorCommandBus_ServosCommandBus.ServosCommandF16Bus.cmdElevator_nd = 0;
    state step_4
      actuatorCommandBus_ServosCommandBus.ServosCommandF16Bus.cmdAileron_nd= 0;
    state EndTest
      stopTest = true;
    (default) -> rollStepInput.Initialize
    rollStepInput.Initialize -> rollStepInput.step_2 : [
        | after(1,tick)
        | ]
    rollStepInput.step_2 -> rollStepInput.step_3 : [
        | after(22,sec)
        | ]
    rollStepInput.step_3 -> rollStepInput.step_1 : [
        | after(10,sec)
        | ]
    rollStepInput.step_1 -> rollStepInput.step_5 : [
        | after(20,sec)
        | ]
    rollStepInput.step_5 -> rollStepInput.step_4 : [
        | after(1,sec)
        | ]
    rollStepInput.step_4 -> rollStepInput.EndTest : [
        | after(10,sec)
        | ]
  state LoopAndBarrelRoll
    state Initialize
      %% Initialize data outputs.
      actuatorCommandBus_controllerArmed = 0;
      actuatorCommandBus_ServosCommandBus.ServosCommandF16Bus.cmdAileron_nd = 0;
      actuatorCommandBus_ServosCommandBus.ServosCommandF16Bus.cmdElevator_nd = 0;
      actuatorCommandBus_ServosCommandBus.ServosCommandF16Bus.cmdRudder_nd = 0;
      actuatorCommandBus_EngineCommandBus.cmdThrottle_unit = 0;
      initialConditionBus = 0;
      environmentBus_EarthEnvironment.gravityScalar_mps2 = 9.80665;
      environmentBus_EarthEnvironment.worldMagneticFieldInNED_nT = zeros(3,1);
      environmentBus_AirEnvironment.airTemperature_K = 0;
      environmentBus_AirEnvironment.airPressure_Pa = 0;
      environmentBus_AirEnvironment.airDensity_kgpm3 = 1.225;
      environmentBus_AirEnvironment.windSpeedInNED_mps = zeros(3,1);
      environmentBus_AirEnvironment.speedOfSound_mps = 0;
      environmentBus_AirEnvironment.windsAloftInNED_mps = zeros(3,1);
      environmentBus_AirEnvironment.gustInNED_mps = zeros(3,1);
      environmentBus_AirEnvironment.turbulenceInNED_mps = zeros(3,1);
      environmentBus_TerrainEnvironment.terrainHeightInNED_m = terrainHeightNED_m;
      stopTest = false;
    state step_2
      actuatorCommandBus_controllerArmed = 1;
      actuatorCommandBus_EngineCommandBus.cmdThrottle_unit = 1;
    state step_3
      actuatorCommandBus_ServosCommandBus.ServosCommandF16Bus.cmdElevator_nd = -0.08;
    state step_1
      actuatorCommandBus_ServosCommandBus.ServosCommandF16Bus.cmdElevator_nd = -0.028;
    state step_5
      actuatorCommandBus_ServosCommandBus.ServosCommandF16Bus.cmdElevator_nd = -1;
    state step_6
      actuatorCommandBus_ServosCommandBus.ServosCommandF16Bus.cmdElevator_nd = 0;
    state EndTest
      stopTest = true;
    (default) -> LoopAndBarrelRoll.Initialize
    LoopAndBarrelRoll.Initialize -> LoopAndBarrelRoll.step_2 : [
        | after(1,tick)
        | ]
    LoopAndBarrelRoll.step_2 -> LoopAndBarrelRoll.step_3 : [
        | after(22,sec)
        | ]
    LoopAndBarrelRoll.step_3 -> LoopAndBarrelRoll.step_1 : [
        | after(10,sec)
        | ]
    LoopAndBarrelRoll.step_5 -> LoopAndBarrelRoll.step_6 : [
        | after(2.5,sec) & vehicleBus.BodyStates.aircraftEulerAngles_rad(2) <0
        | ]
    LoopAndBarrelRoll.step_6 -> LoopAndBarrelRoll.EndTest : [
        | after(10,sec)
        | ]
    LoopAndBarrelRoll.step_1 -> LoopAndBarrelRoll.step_5 : [
        | after(20,sec)
        | ]
  (default) -> Scenario_1 [order 1] : [Active_Scenario_Index == 1]
  (default) -> SameAsVehiclePlantHarness [order 2] : [Active_Scenario_Index == 2]
  (default) -> MaxAirspeedTest [order 3] : [Active_Scenario_Index == 3]
  (default) -> TakeoffLevelFlight [order 4] : [Active_Scenario_Index == 4]
  (default) -> pitchTest [order 5] : [Active_Scenario_Index == 5]
  (default) -> rollTest [order 6] : [Active_Scenario_Index == 6]
  (default) -> pitchStepInput [order 7] : [Active_Scenario_Index == 7]
  (default) -> rollStepInput [order 8] : [Active_Scenario_Index == 8]
  (default) -> LoopAndBarrelRoll [order 9] : {assert(Active_Scenario_Index == 9,'The value of Scenario Parameter ''Active_Scenario_Index'' is not valid. Use the index of the scenario to specify it.')}
  data: vehicleBus input Bus: VehicleBus size=[1]; actuatorCommandBus_controllerArmed output double size=[1]; actuatorCommandBus_ServosCommandBus output Bus: ServosCommandBus size=[1]; actuatorCommandBus_EngineCommandBus output Bus: EngineCommandBus size=[1]; initialConditionBus output double size=[1]; environmentBus_EarthEnvironment output Bus: EarthEnvironmentBus size=[1]; environmentBus_AirEnvironment output Bus: AirEnvironmentBus size=[1]; environmentBus_TerrainEnvironment output Bus: TerrainEnvironmentBus size=[1]; stopTest output; Active_Scenario_Index parameter =1; terrainHeightNED_m parameter
